simulink model "cont_100"  (Simulink 10.0)
settings: Solver=FixedStepDiscrete  StartTime=0.0  StopTime=inf  FixedStep=1  RelTol=1e-3  EnableMultiTasking=on
settings Model: Creator=prof. G. Celentano  LastModifiedBy=giuseppericcio
settings DataIOCC: LimitDataPoints=on  SignalLoggingSaveFormat=ModelDataLogs  SignalLoggingName=sigsOut
settings OptimizationCC: BlockReduction=off  BooleanDataType=off  ExpressionDepthLimit=2147483647
settings DebuggingCC: SaveWithParameterizedLinksMsg=none  SignalResolutionControl=TryResolveAllWithWarning  MultiTaskDSMMsg=warning  MultiTaskCondExecSysMsg=none  FcnCallInpInsideContextMsg=warning  StateNameClashWarn=warning
settings HardwareCC: ProdIntDivRoundTo=Zero  ProdEndianess=LittleEndian  ProdHWDeviceType=Generic->32-bit x86 compatible  TargetUnknown=on
settings RTWCC: SystemTargetFile=rtwin.tlc  TemplateMakefile=rtwintmf  RTWCompilerOptimization=on
settings TargetCC: TargetLibSuffix=_rtwin.lib  TargetPreCompLibLocation=C:\Program Files (x86)\MATLAB\R2008b\toolbox\rtw\targets\rtwin\lib  GeneratePreprocessorConditionals=Use local settings  PreserveStateflowLocalDataDimensions=off
settings CustomProperty: DataType=string

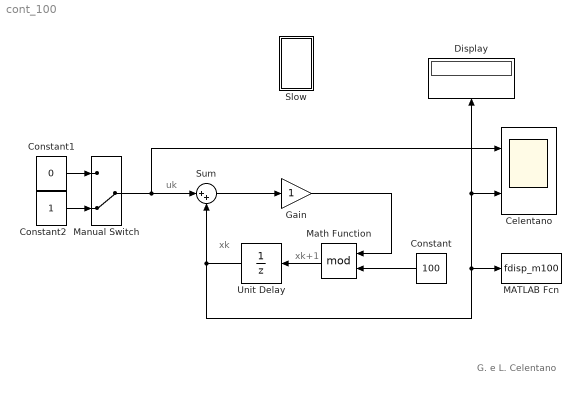
== system cont_100 ==
  note: xk+1
  note: xk
  note: uk
  note: G. e L. Celentano
  Celentano : Scope  NumInputPorts=2
  Constant : Constant  Value=100
  Constant1 : Constant  Value=0
  Constant2 : Constant
  Display : Display
  Gain : Gain  SaturateOnIntegerOverflow=on  OutDataTypeStr=Inherit: Same as input  ParamDataTypeStr=Inherit: Same as input
  MATLAB Fcn : MATLABFcn  MATLABFcn=fdisp_m100
  Manual Switch : ManualSwitch  CurrentSetting=0
  Math Function : Math  Operator=mod  SaturateOnIntegerOverflow=on
  Slow : Subsystem
      mask Display: plot([0 1],[0 1])
  Sum : Sum  Inputs=|++  SaturateOnIntegerOverflow=on
  Unit Delay : UnitDelay
  wires:
  Manual Switch/1 -> Celentano/1, Sum/1
  Sum/1 -> Gain/1
  Gain/1 -> Math Function/1
  Unit Delay/1 -> Sum/2, Display/1, Celentano/2, MATLAB Fcn/1
  Math Function/1 -> Unit Delay/1
  Constant/1 -> Math Function/2
  Constant1/1 -> Manual Switch/1
  Constant2/1 -> Manual Switch/2

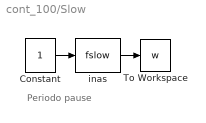
== system cont_100/Slow ==
  note: Periodo
      | pause
  Constant : Constant
  To Workspace : ToWorkspace  VariableName=w  SampleTime=-1
  inas : MATLABFcn  MATLABFcn=fslow
  wires:
  Constant/1 -> inas/1
  inas/1 -> To Workspace/1
